simulink model "LQR_Example2"  (R2014a)
settings: Solver=ode45  StartTime=0.0  StopTime=10.0  RelTol=1e-3
InitFcn:
  | load('Matrix.mat')
  | 
  | % % 제어기 설정 %
  | Q1 = 5;        % Lateral Offset 의 가중치
  | Q2 = 30;        % Drift Angle의 가중치
  | R =  250;       % Steering Angle의 가중치
  | PL = [-50-50i,-50+50i,-30,-20]; % Observer 극점
  | 
  | [K,L] = sfGain(Q1,Q2,R,PL);
values from neighbouring files (symbols this model uses):
  A = [2 3;-1 4]    [LQR_Example.m]
  B = [0;1]    [LQR_Example.m]
  K = lqr(A,B,Q,R)    [LQR_Example.m]
undefined symbols (not defined in the file or in its folder): L
settings Model: Creator=IVDL  LastModifiedBy=user
settings OptimizationCC: SimCompilerOptimization=off
settings DebuggingCC: UnderspecifiedInitializationDetection=Classic  FrameProcessingCompatibilityMsg=error  StateNameClashWarn=warning
settings RTWCC: RTWCompilerOptimization=off
settings ConfigComp: CovMetricSettings=dw  CovHtmlReporting=on  CovSaveCumulativeToWorkspaceVar=on  CovSaveSingleToWorkspaceVar=on  CovModelRefEnable=Off  CovExternalEMLEnable=off

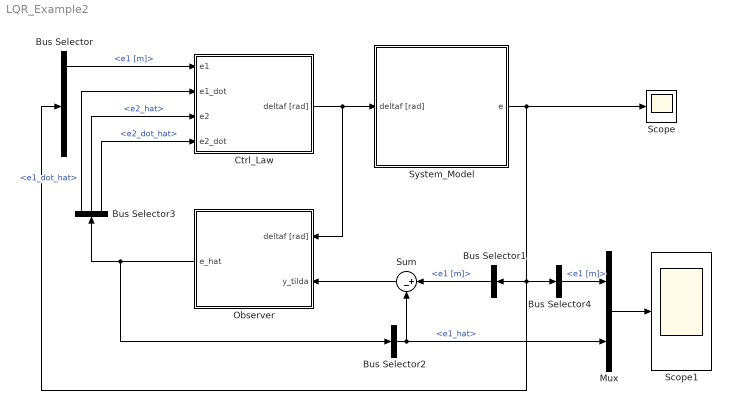
== system LQR_Example2 ==
  Bus Selector : BusSelector  OutputSignals=e1 [m],e1_dot [m/s],e2 [rad],e2_dot [rad/s]
  Bus Selector1 : BusSelector  OutputSignals=e1 [m]
  Bus Selector2 : BusSelector  OutputSignals=e1_hat
  Bus Selector3 : BusSelector  OutputSignals=e1_dot_hat,e2_hat,e2_dot_hat
  Bus Selector4 : BusSelector  OutputSignals=e1 [m]
  Ctrl_Law : Subsystem
  Mux : Mux  Inputs=2
  Observer : Subsystem
  Scope : Scope
  Scope1 : Scope
  Sum : Sum  Inputs=|+-
  System_Model : Subsystem
  wires:
  System_Model/1(e) -> Scope/1, Bus Selector4/1, Bus Selector/1, Bus Selector1/1
  Ctrl_Law/1(deltaf [rad]) -> System_Model/1(deltaf [rad]), Observer/1(deltaf [rad])
  Bus Selector/1 -> Ctrl_Law/1(e1)  "<e1 [m]>"
  Observer/1(e_hat) -> Bus Selector2/1, Bus Selector3/1
  Sum/1 -> Observer/2(y_tilda)
  Bus Selector1/1 -> Sum/1  "<e1 [m]>"
  Bus Selector2/1 -> Mux/2, Sum/2  "<e1_hat>"
  Bus Selector4/1 -> Mux/1  "<e1 [m]>"
  Mux/1 -> Scope1/1
  Bus Selector3/3 -> Ctrl_Law/4(e2_dot)  "<e2_dot_hat>"
  Bus Selector3/2 -> Ctrl_Law/3(e2)  "<e2_hat>"
  Bus Selector3/1 -> Ctrl_Law/2(e1_dot)  "<e1_dot_hat>"

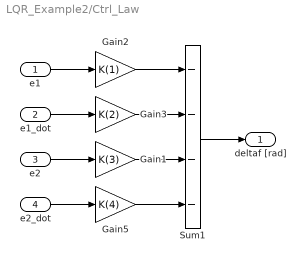
== system LQR_Example2/Ctrl_Law ==
  e1 : Inport
  e1_dot : Inport  Port=2
  e2 : Inport  Port=3
  e2_dot : Inport  Port=4
  Gain1 : Gain  Gain=K(3)
  Gain2 : Gain  Gain=K(1)
  Gain3 : Gain  Gain=K(2)
  Gain5 : Gain  Gain=K(4)
  Sum1 : Sum  Inputs=----
  deltaf [rad] : Outport
  wires:
  Sum1/1 -> deltaf [rad]/1
  Gain2/1 -> Sum1/1
  Gain5/1 -> Sum1/4
  e2_dot/1 -> Gain5/1
  e1_dot/1 -> Gain3/1
  Gain3/1 -> Sum1/2
  Gain1/1 -> Sum1/3
  e1/1 -> Gain2/1
  e2/1 -> Gain1/1

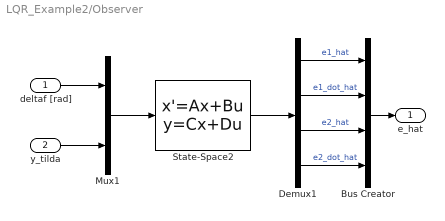
== system LQR_Example2/Observer ==
  deltaf [rad] : Inport
  y_tilda : Inport  Port=2
  Bus Creator : BusCreator
  Demux1 : Demux
  Mux1 : Mux  Inputs=2
  State-Space2 : StateSpace  A=A  B=[B L']  C=diag([1 1 1 1])  D=zeros(4,2)  X0=0  ContinuousStateAttributes={'e1','e1_dot','e2','e2_dot'}
  e_hat : Outport
  wires:
  Mux1/1 -> State-Space2/1
  deltaf [rad]/1 -> Mux1/1
  Demux1/4 -> Bus Creator/4  "e2_dot_hat"
  Demux1/2 -> Bus Creator/2  "e1_dot_hat"
  Demux1/3 -> Bus Creator/3  "e2_hat"
  y_tilda/1 -> Mux1/2
  State-Space2/1 -> Demux1/1
  Demux1/1 -> Bus Creator/1  "e1_hat"
  Bus Creator/1 -> e_hat/1

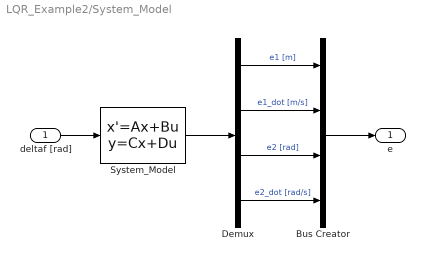
== system LQR_Example2/System_Model ==
  deltaf [rad] : Inport
  Bus Creator : BusCreator
  Demux : Demux
  System_Model : StateSpace  A=A  B=B  C=diag([1 1 1 1])  D=[0;0;0;0]  X0=[3.6/2, 0, 10*pi/180, 0]
  e : Outport
  wires:
  System_Model/1 -> Demux/1
  deltaf [rad]/1 -> System_Model/1
  Demux/2 -> Bus Creator/2  "e1_dot [m/s]"
  Demux/3 -> Bus Creator/3  "e2 [rad]"
  Demux/4 -> Bus Creator/4  "e2_dot [rad/s]"
  Demux/1 -> Bus Creator/1  "e1 [m]"
  Bus Creator/1 -> e/1
